simulink model "Bat_Cool_Cabin_Heat"  (R2021b)
settings: Solver=VariableStepAuto  StartTime=0.0  StopTime=1000  RelTol=1e-3
libraries: fl_lib x21, nesl_utility x6
settings Model: Creator=lenovo  LastModifiedBy=lenovo

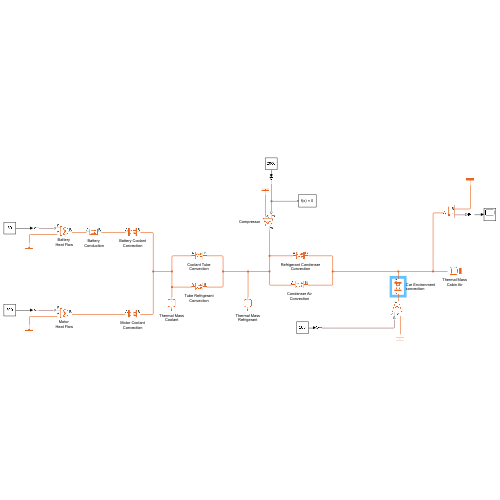
[thumbnail: Simulink's stored preview of the top-level diagram]
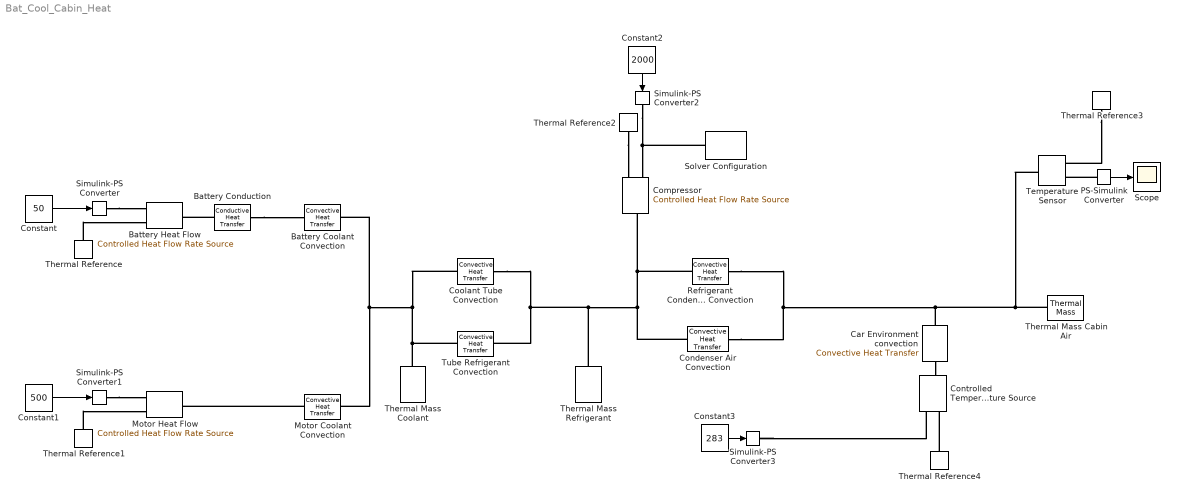
== system Bat_Cool_Cabin_Heat ==
  Battery Conduction : fl_lib/Thermal/Thermal Elements/Conductive Heat Transfer  area=5.33 m^2  thickness=0.018 m  th_cond=15 W/(m*K)  T_specify=off  T_priority=None  T=0 K  T_nominal_specify=off  T_nominal_unit=K  T_nominal_value=1  Q_specify=on  Q_priority=High  Q=50 W  Q_nominal_specify=off  Q_nominal_unit=W  Q_nominal_value=1
  Battery Heat Flow : fl_lib/Thermal/Thermal Sources/Controlled Heat Flow Rate Source
  Battery Coolant Convection : fl_lib/Thermal/Thermal Elements/Convective Heat Transfer  area=5.33 m^2  heat_tr_coeff=1900 W/(m^2*K)  T_specify=off  T_priority=None  T=0 K  T_nominal_specify=off  T_nominal_unit=K  T_nominal_value=1  Q_specify=off  Q_priority=None  Q=0 W  Q_nominal_specify=off  Q_nominal_unit=W  Q_nominal_value=1
  Car Environment convection : fl_lib/Thermal/Thermal Elements/Convective Heat Transfer  area=18 m^2  heat_tr_coeff=8 W/(m^2*K)  T_specify=off  T_priority=None  T=0 K  T_nominal_specify=off  T_nominal_unit=K  T_nominal_value=1  Q_specify=off  Q_priority=None  Q=0 W  Q_nominal_specify=off  Q_nominal_unit=W  Q_nominal_value=1
  Compressor : fl_lib/Thermal/Thermal Sources/Controlled Heat Flow Rate Source
  Condenser Air Convection : fl_lib/Thermal/Thermal Elements/Convective Heat Transfer  area=0.25 m^2  heat_tr_coeff=55 W/(m^2*K)  T_specify=off  T_priority=None  T=0 K  T_nominal_specify=off  T_nominal_unit=K  T_nominal_value=1  Q_specify=off  Q_priority=None  Q=0 W  Q_nominal_specify=off  Q_nominal_unit=W  Q_nominal_value=1
  Constant : Constant  Value=50
  Constant1 : Constant  Value=500
  Constant2 : Constant  Value=2000
  Constant3 : Constant  Value=283
  Controlled Temperature Source : fl_lib/Thermal/Thermal Sources/Controlled Temperature Source
  Coolant Tube Convection : fl_lib/Thermal/Thermal Elements/Convective Heat Transfer  area=0.02 m^2  heat_tr_coeff=6900 W/(m^2*K)  T_specify=off  T_priority=None  T=0 K  T_nominal_specify=off  T_nominal_unit=K  T_nominal_value=1  Q_specify=off  Q_priority=None  Q=0 W  Q_nominal_specify=off  Q_nominal_unit=W  Q_nominal_value=1
  Motor Heat Flow : fl_lib/Thermal/Thermal Sources/Controlled Heat Flow Rate Source
  Motor Coolant Convection : fl_lib/Thermal/Thermal Elements/Convective Heat Transfer  area=0.02 m^2  heat_tr_coeff=1800 W/(m^2*K)  T_specify=off  T_priority=None  T=0 K  T_nominal_specify=off  T_nominal_unit=K  T_nominal_value=1  Q_specify=off  Q_priority=None  Q=0 W  Q_nominal_specify=off  Q_nominal_unit=W  Q_nominal_value=1
  PS-Simulink Converter : nesl_utility/PS-Simulink Converter  PhysicalDomain=network_engine_domain  SubClassName=ps_output  LeftPortType=input  RightPortType=output  PseudoPeriodic=off  Frequencies=[]  Unit=inherit  AffineConversion=off
      settings: SourceProductBaseCode=PW,SS
  Refrigerant Condenser Convection : fl_lib/Thermal/Thermal Elements/Convective Heat Transfer  area=0.25 m^2  heat_tr_coeff=1065 W/(m^2*K)  T_specify=off  T_priority=None  T=0 K  T_nominal_specify=off  T_nominal_unit=K  T_nominal_value=1  Q_specify=off  Q_priority=None  Q=0 W  Q_nominal_specify=off  Q_nominal_unit=W  Q_nominal_value=1
  Scope : Scope
  Simulink-PS Converter{,1..3} (4 alike) : nesl_utility/Simulink-PS Converter  PhysicalDomain=network_engine_domain  SubClassName=ps_input  LeftPortType=input  RightPortType=output  PseudoPeriodic=off  Frequencies=[]  NoiseDistribution=none  NoiseParameters=[]  Unit=1  AffineConversion=off  FilteringAndDerivatives=provide  SimscapeFilterOrder=1  InputFilterTimeConstant=0.001  UdotUserProvided=0
      settings: SourceProductBaseCode=PW,SS
  Solver Configuration : nesl_utility/Solver Configuration  PhysicalDomain=network_engine_domain  SubClassName=solver  LeftPortType=input  RightPortType=generic  Tones=[]  Harmonics=[]  SimulateNoise=off  Profile=off  UseLocalSampling=off  EnableSwitchedLinearOptims=on  FrequencyDomain=off  UseCCode=off  RelTol=0.001  AbsTol=1e-06  MinStep=1e-09  ToWorkspace=off  RevertToSquareIcSolve=off  NumHomotopyIterations=100  PhasorMode=off  PhasorModeNumHarmonics=1  DoDC=off  ResidualTolerance=1e-09  UseLocalSolver=off  LocalSolverChoice=NE_BACKWARD_EULER_ADVANCER  LocalSolverSampleTime=0.001  DoFixedCost=off  MaxNonlinIter=3  MaxModeIter=2  ComputeImpulses=off  ImpulseIterations=2  LinearAlgebra=auto  EquationFormulation=NE_TIME_EF  DelaysMemoryBudget=1024  AutomaticFiltering=on  FilteringTimeConstant=0.001  PartitionStorageMethod=AS_NEEDED  PartitionMemoryBudget=1024  PartitionMethod=ROBUST
      settings: SourceProductBaseCode=PW,SS
  Temperature Sensor : fl_lib/Thermal/Thermal Sensors/Temperature Sensor
  Thermal Mass Cabin Air : fl_lib/Thermal/Thermal Elements/Thermal Mass  mass=3.6 kg  sp_heat=1005 J/(K*kg)  T_specify=on  T_priority=High  T=283 K  T_nominal_specify=off  T_nominal_unit=K  T_nominal_value=1  Q_specify=off  Q_priority=None  Q=0 W  Q_nominal_specify=off  Q_nominal_unit=W  Q_nominal_value=1
  Thermal Mass Coolant : fl_lib/Thermal/Thermal Elements/Thermal Mass  mass=20 kg  sp_heat=3500 J/(K*kg)  T_specify=off  T_priority=High  T=300 K  T_nominal_specify=off  T_nominal_unit=K  T_nominal_value=1  Q_specify=off  Q_priority=None  Q=0 W  Q_nominal_specify=off  Q_nominal_unit=W  Q_nominal_value=1
  Thermal Mass Refrigerant : fl_lib/Thermal/Thermal Elements/Thermal Mass  mass=1 kg  sp_heat=797 J/(K*kg)  T_specify=off  T_priority=High  T=300 K  T_nominal_specify=off  T_nominal_unit=K  T_nominal_value=1  Q_specify=off  Q_priority=None  Q=0 W  Q_nominal_specify=off  Q_nominal_unit=W  Q_nominal_value=1
  Thermal Reference{,1..4} (5 alike) : fl_lib/Thermal/Thermal Elements/Thermal Reference
  Tube Refrigerant Convection : fl_lib/Thermal/Thermal Elements/Convective Heat Transfer  area=0.02 m^2  heat_tr_coeff=1060 W/(m^2*K)  T_specify=off  T_priority=None  T=0 K  T_nominal_specify=off  T_nominal_unit=K  T_nominal_value=1  Q_specify=off  Q_priority=None  Q=0 W  Q_nominal_specify=off  Q_nominal_unit=W  Q_nominal_value=1
  wires:
  Constant/1 -> Simulink-PS Converter/1
  Constant1/1 -> Simulink-PS Converter1/1
  Constant2/1 -> Simulink-PS Converter2/1
  PS-Simulink Converter/1 -> Scope/1
  Constant3/1 -> Simulink-PS Converter3/1
  connections:
  Simulink-PS Converter/RConn1 -- Battery Heat Flow/RConn1
  Thermal Reference/LConn1 -- Battery Heat Flow/RConn2
  Battery Conduction/LConn1 -- Battery Heat Flow/LConn1
  Thermal Reference1/LConn1 -- Motor Heat Flow/RConn2
  Simulink-PS Converter1/RConn1 -- Motor Heat Flow/RConn1
  Simulink-PS Converter2/RConn1 -- Solver Configuration/RConn1 -- Compressor/RConn1
  Thermal Reference2/LConn1 -- Compressor/RConn2
  Battery Conduction/RConn1 -- Battery Coolant Convection/LConn1
  Thermal Mass Refrigerant/LConn1 -- Tube Refrigerant Convection/RConn1 -- Coolant Tube Convection/RConn1 -- Refrigerant Condenser Convection/LConn1 -- Compressor/LConn1 -- Condenser Air Convection/LConn1
  Motor Coolant Convection/LConn1 -- Motor Heat Flow/LConn1
  Thermal Mass Coolant/LConn1 -- Coolant Tube Convection/LConn1 -- Battery Coolant Convection/RConn1 -- Motor Coolant Convection/RConn1 -- Tube Refrigerant Convection/LConn1
  Thermal Mass Cabin Air/LConn1 -- Condenser Air Convection/RConn1 -- Refrigerant Condenser Convection/RConn1 -- Car Environment convection/RConn1 -- Temperature Sensor/LConn1
  Thermal Reference3/LConn1 -- Temperature Sensor/RConn1
  PS-Simulink Converter/LConn1 -- Temperature Sensor/RConn2
  Simulink-PS Converter3/RConn1 -- Controlled Temperature Source/RConn1
  Thermal Reference4/LConn1 -- Controlled Temperature Source/RConn2
  Car Environment convection/LConn1 -- Controlled Temperature Source/LConn1
